simulink model "signala_simulink_vid"  (R2020a)
settings: Solver=FixedStepDiscrete  StartTime=0  StopTime=6  FixedStep=0.01  RelTol=1e-3
values from neighbouring files (symbols this model uses):
  signala_rokturis = @(t) signals(t)    [nosledzosaisLabDarbs_VladimirsFedorovics.m]
undefined symbols (not defined in the file or in its folder): DiscIntNeverNeededParam
settings Model: Creator=Vladimirs  LastModifiedBy=Vladimirs

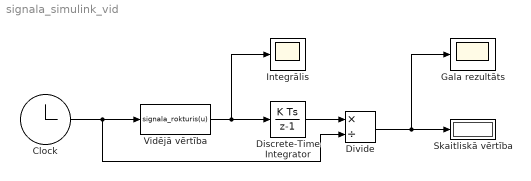
== system signala_simulink_vid ==
  Clock : Clock
  Discrete-Time Integrator : DiscreteIntegrator  SampleTime=-1  ICPrevOutput=DiscIntNeverNeededParam  ICPrevScaledInput=DiscIntNeverNeededParam
  Divide : Product  Inputs=*/
  Gala rezultāts : Scope
  Integrālis : Scope
  Skaitliskā vērtība : Display
  Vidējā vērtība : MATLABFcn  MATLABFcn=signala_rokturis(u)
  wires:
  Clock/1 -> Divide/2, Vidējā vērtība/1
  Vidējā vērtība/1 -> Integrālis/1, Discrete-Time Integrator/1
  Discrete-Time Integrator/1 -> Divide/1
  Divide/1 -> Gala rezultāts/1, Skaitliskā vērtība/1
